simulink model "Segway_Lineare_nuovip"  (R2023b)
settings: Solver=VariableStepAuto  StartTime=0.0  StopTime=50  RelTol=1e-3
values from neighbouring files (symbols this model uses):
  Gtot = minreal(Gtot)    [CSI1_Segway_LQG_nuovip.m]
  K_LQG = -lqgreg(kest, Klqr)    [CSI1_Segway_LQG_nuovip.m]
undefined symbols (not defined in the file or in its folder): K_DK, K_MS
settings Model: Creator=dario  LastModifiedBy=dario

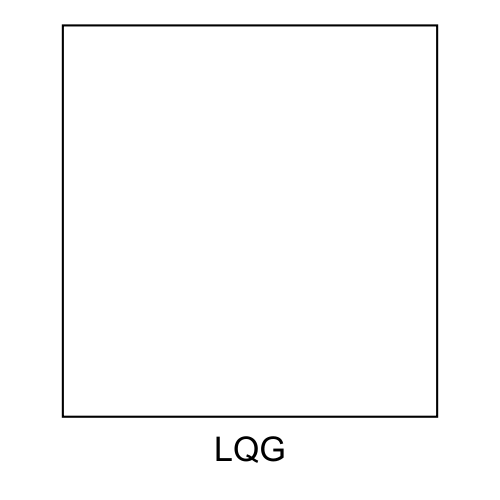
[thumbnail: Simulink's stored preview of the top-level diagram]
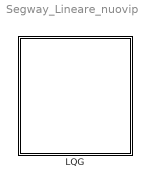
== system Segway_Lineare_nuovip ==
  LQG : Subsystem

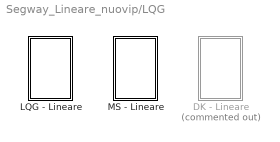
== system Segway_Lineare_nuovip/LQG ==
  DK - Lineare : Subsystem  Commented=on
  LQG - Lineare : Subsystem
  MS - Lineare : Subsystem

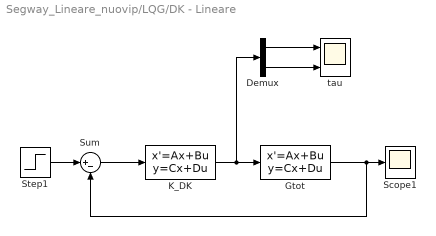
== system Segway_Lineare_nuovip/LQG/DK - Lineare ==
  Demux : Demux  Outputs=2
  Gtot : StateSpace  A=Gtot.A  B=Gtot.B  C=Gtot.C  D=Gtot.D  InitialCondition=0
  K_DK : StateSpace  A=K_DK.A  B=K_DK.B  C=K_DK.C  D=K_DK.D  InitialCondition=0
  Scope1 : Scope
  Step1 : Step  Before=[0 0 0]'  After=[1 0 0]'  SampleTime=0
  Sum : Sum  Inputs=|+-
  tau : Scope  NumInputPorts=2
  wires:
  K_DK/1 -> Demux/1, Gtot/1
  Gtot/1 -> Sum/2, Scope1/1
  Demux/2 -> tau/2
  Sum/1 -> K_DK/1
  Demux/1 -> tau/1
  Step1/1 -> Sum/1

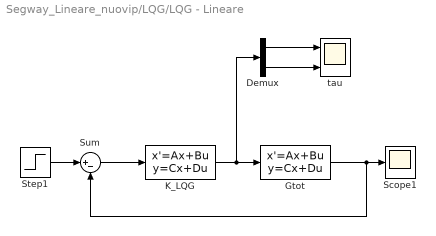
== system Segway_Lineare_nuovip/LQG/LQG - Lineare ==
  Demux : Demux  Outputs=2
  Gtot : StateSpace  A=Gtot.A  B=Gtot.B  C=Gtot.C  D=Gtot.D  InitialCondition=0
  K_LQG : StateSpace  A=K_LQG.A  B=K_LQG.B  C=K_LQG.C  D=K_LQG.D  InitialCondition=0
  Scope1 : Scope
  Step1 : Step  Before=[0 0 0]'  After=[1 0 0]'  SampleTime=0
  Sum : Sum  Inputs=|+-
  tau : Scope  NumInputPorts=2
  wires:
  K_LQG/1 -> Demux/1, Gtot/1
  Gtot/1 -> Sum/2, Scope1/1
  Demux/2 -> tau/2
  Sum/1 -> K_LQG/1
  Demux/1 -> tau/1
  Step1/1 -> Sum/1

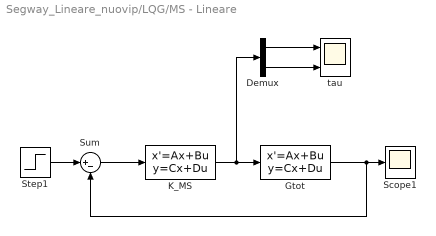
== system Segway_Lineare_nuovip/LQG/MS - Lineare ==
  Demux : Demux  Outputs=2
  Gtot : StateSpace  A=Gtot.A  B=Gtot.B  C=Gtot.C  D=Gtot.D  InitialCondition=0
  K_MS : StateSpace  A=K_MS.A  B=K_MS.B  C=K_MS.C  D=K_MS.D  InitialCondition=0
  Scope1 : Scope
  Step1 : Step  Before=[0 0 0]'  After=[1 0 0]'  SampleTime=0
  Sum : Sum  Inputs=|+-
  tau : Scope  NumInputPorts=2
  wires:
  Step1/1 -> Sum/1
  Demux/1 -> tau/1
  Sum/1 -> K_MS/1
  Demux/2 -> tau/2
  Gtot/1 -> Scope1/1, Sum/2
  K_MS/1 -> Gtot/1, Demux/1
